simulink library "hmi_udp_lib"  (Simulink 8.2)
settings: Solver=ode1  StartTime=0.0  StopTime=Inf  FixedStep=0.001  RelTol=1e-3
PostLoadFcn:
  | , if any(exist('dsrtsu_mdlpostloadfcn', 'file') == [2, 3, 6]), try dsrtsu_mdlpostloadfcn('Execute', bdroot); catch fprintf('Error in PostLoadFcn (dsrtsu_mdlpostloadfcn) for model "%s":\n %s\n', bdroot, lasterr); end, end,
undefined symbols (not defined in the file): XXX
libraries: rtiethernetudplib x2, parse_utils x1
settings Model: DSRTSU_INTERNAL_RTI_VER=450  DSRTSU_INTERNAL_RTI_TYPE=rti1401  DSRTSU_INTERNAL_RTIFPGA=40  Creator=rushk1  LastModifiedBy=rushk1

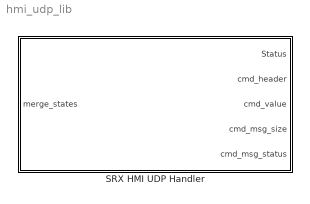
== system hmi_udp_lib ==
  SRX HMI UDP Handler : Subsystem

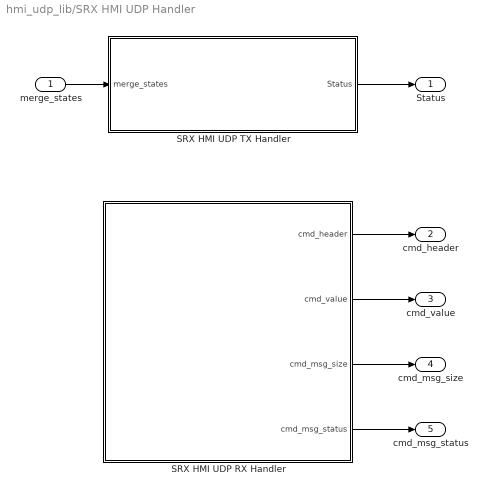
== system hmi_udp_lib/SRX HMI UDP Handler ==
  merge_states : Inport
  SRX HMI UDP RX Handler : Subsystem
  SRX HMI UDP TX Handler : Subsystem
  Status : Outport
  cmd_header : Outport  Port=2
  cmd_value : Outport  Port=3
  cmd_msg_size : Outport  Port=4
  cmd_msg_status : Outport  Port=5
  wires:
  SRX HMI UDP TX Handler/1(Status) -> Status/1
  merge_states/1 -> SRX HMI UDP TX Handler/1(merge_states)
  SRX HMI UDP RX Handler/4(cmd_msg_status) -> cmd_msg_status/1
  SRX HMI UDP RX Handler/3(cmd_msg_size) -> cmd_msg_size/1
  SRX HMI UDP RX Handler/2(cmd_value) -> cmd_value/1
  SRX HMI UDP RX Handler/1(cmd_header) -> cmd_header/1

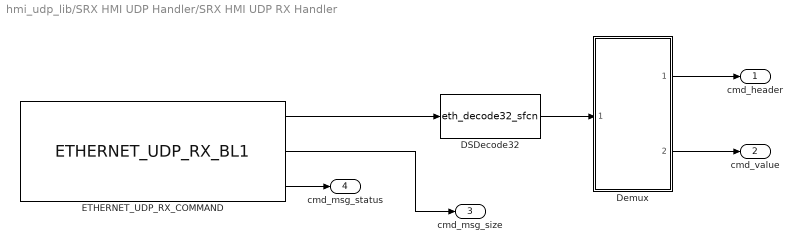
== system hmi_udp_lib/SRX HMI UDP Handler/SRX HMI UDP RX Handler ==
  "DSDecode32 " : S-Function  FunctionName=eth_decode32_sfcn  Parameters=byteordering,offset,auto_offset,datatype,one_datatype,sampletime  EnableBusSupport=off  mask(DSDecode32){byteordering=big endian (Motorola), offset=[0], auto_offset=on, datatype=[3,3], one_datatype=off, sampletime=-1}
      mask prompts: byteordering "Byte ordering:"; offset "Offset (bytes):"; auto_offset "Auto offset"; one_datatype "One datatype only"
      mask help:
      | Converts a 32bit WORD input data stream into the specified datatypes on the output port.
      |
      | Datatype Codes:
      | BOOLEAN:  1   //   INT8      :  2    //   UINT8    :  3
      | INT16       :  4   //   UINT16 :  5    //   INT32     :  6
      | UINT32    :  7   //   FLOAT   :  8    //   DOUBLE:  9
      mask Help:
      | The 'DSDecode32' block allows to decode an UInt32 vector containing encoded elements of various data types to an output vector of double values. It is intended to use this block in conjunction with the 'DS4504_ETH_Receive' block which delivers this format as data output. Data received from the Ethernet via the 'DS4504_ETH_Receive' block is performed in Intel byte order ('Little Endian').
      | 
      | <br>
      | <br>
      | 
      | <h2>Parameters</h2>
      | <br>
      | <br>
      | 
      | <b>Byte ordering (only relevant for offline simulation)</b>
      | <br>
      | <blockquote>
      | The byte order of the input vector has to be specified. In case of running a real-time application the appropriate byte order (Motorola for DS1005 and Intel for DS1006) is selected automatically. Therefore the byte order setting has no influence on the online simulation.
      | </blockquote>
      | <br>
      | 
      | <b>Offset (bytes)</b>
      | <br>
      | <blockquote>
      | This is for defining a vector of offsets which specifies the position of each element within the input vector. The offsets must be entered as an array (e.g. [1 10 . 50 54] ) using the same order as for the corresponding data type vector (see (4)). This option is useful if you have gaps between adjacent elements.
      | </blockquote>
      | <br>
      | 
      | <b>Auto offset</b>
      | <br>
      | <blockquote>
      | When activating this checkbox parameter, the edit field 'Offset' is disabled and the byte offsets in the input vector are calculated automatically concerning the specified data types (no gaps presupposed). Any previous setting in the offset vector would be ignored.
      | </blockquote>
      | <br>
      | 
      | <b>Datatype</b>
      | <br>
      | <blockquote>
      | This is for defining a vector of data types which specifies the type for each element in the input vector. Supported data types are Boolean, Int8, UInt8, Int16, UInt16, Int32, UInt32, Float and Double, which are determined by using the corresponding data type codes shown in the following table:
      | <br>
      | <br>
      | <table BORDER=1 ALIGN="center">
      | <TR>
      | <TH WIDTH=20%>Data type</TH>
      | <TH WIDTH=20%>Data type code</TH>
      | <TH WIDTH=20%>Length in bytes</TH>
      | </TR>
      | <TR><TD>Boolean</TD><TD ALIGN="center">1</TD><TD ALIGN="center">1</TD></TR>
      | <TR><TD>Int8</TD><TD ALIGN="center">2</TD><TD ALIGN="center">1</TD></TR>
      | <TR><TD>Uint8</TD><TD ALIGN="center">3</TD><TD ALIGN="center">1</TD></TR>
      | <TR><TD>Int16</TD><TD ALIGN="center">4</TD><TD ALIGN="center">2</TD></TR>
      | <TR><TD>Uint16</TD><TD ALIGN="center">5</TD><TD ALIGN="center">2</TD></TR>
      | <TR><TD>Int32</TD><TD ALIGN="center">6</TD><TD ALIGN="center">4</TD></TR>
      | <TR><TD>Uint32</TD><TD ALIGN="center">7</TD><TD ALIGN="center">4</TD></TR>
      | <TR><TD>Float</TD><TD ALIGN="center">8</TD><TD ALIGN="center">4</TD></TR>
      | <TR><TD>Double</TD><TD ALIGN="center">9</TD><TD ALIGN="center">8</TD></TR>
      | </TABLE>
      | </blockquote>
      | <br>
      | 
      | <b>One datatype only</b>
      | <br>
      | <blockquote>
      | This option is useful if all elements of the input vector have the same data type. If the checkbox is activated the first element of the data type vector specifies the data type to be used. In this case it is naturally sufficient to enter only one number which applies for the complete input vector.
      | </blockquote>
      | <br>
      | 
      | <b>Sample time</b>
      | <br>
      | <blockquote>
      | The desired sample time for this block has to be entered here. Alternatively it can be  inherited from the Simulink model by using '-1'.
      | </blockquote>
      | <br>
      mask TypeOptions byteordering: big endian (Motorola) | little endian (Intel)
      mask Display: text(0.5,0.5,'DSDecode32','HorizontalAlignment','center')
  Demux : Subsystem
  ETHERNET_UDP_RX_COMMAND : rtiethernetudplib/ETHERNET_UDP_RX_BL1  InterfaceName=NOT SPECIFIED  BoardType=ETH Type 1  ModuleNo=1  ChannelNo=1  SocketNo=4  MaxMessageSize=5  LocalSocket=XXX.XXX.XXX.XXX:5000  RemoteSocket=XXX.XXX.XXX.XXX:5000  DSProperties=struct('RTI',struct('Version',uint32(1),'BlockType',struct('isSLSource',uint8(1),'isSLSink',uint8(0),'isHWSource',uint8(0),'isHWSink',uint8(1),'isSetup',uint8(0),'isInline',uint8(1),'isNonInline',uint8(1),'isInterrupt',uint8(0),'isChannelwise',uint8(1)),'IOBoardType','DSETHERNETUDP','UnitType','ETHUDP','Identifier','RX','DialogType','SL','BlockSet','RTIETHERNETUDP','SlaveProcessor','NONE'))  RTIBlockInterface=struct('OutputPortsWidth',int32([1 1 1]),'OutputPortsActive',[1 1 1],'OutputPortsName',{{'Data',['Message Size'],'Status'}},'OutputPortsDataType',{{'SS_UINT32','SS_INT32','SS_BOOLEAN'}},'BlockDisplay',{{['Ethernet UDP Receive\nBoard Type: ETH Type 1\nModule: 1\nSocket: 4\nMaximum Message Size: 5'],'center'}},'IconTransparency','on','InitLevel',3,'BlockName',struct('Token',{{'ETHERNET_UDP_RX_BL1'}}),'MaskDescription',['To receive messages from the Ethernet UDP interface.'])  RTIBlockParameters=struct('InterfaceName',{{['NOT SPECIFIED'],'OFF',[]}},'BoardType',{{1,'OFF',[]}},'ModuleNo',{{1,'OFF',[1 16]}},'ChannelNo',{{1,'OFF',[1 2]}},'SocketNo',{{4,'OFF',[1 4]}},'MaxMessageSize',{{5,'ON',[1 1472]}},'LocalSocket',{{'XXX.XXX.XXX.XXX:5000','OFF',[]}},'RemoteSocket',{{'XXX.XXX.XXX.XXX:5000','OFF',[]}})  RTISFcnParameters=struct('InterfaceName','char','BoardType','double','ModuleNo','double','ChannelNo','double','SocketNo','double','MaxMessageSize','double','LocalSocket','char','RemoteSocket','char')  RTIBlockParaDefault=struct('InterfaceName','rti_ethernet_interface_name','BoardType',1,'ModuleNo',1,'ChannelNo',1,'SocketNo',1,'MaxMessageSize',625,'LocalSocket','XXX.XXX.XXX.XXX:5000','RemoteSocket','XXX.XXX.XXX.XXX:5000')
  cmd_header : Outport
  cmd_value : Outport  Port=2
  cmd_msg_size : Outport  Port=3
  cmd_msg_status : Outport  Port=4
  wires:
  ETHERNET_UDP_RX_COMMAND/1 -> "DSDecode32 "/1
  ETHERNET_UDP_RX_COMMAND/3 -> cmd_msg_status/1
  ETHERNET_UDP_RX_COMMAND/2 -> cmd_msg_size/1
  "DSDecode32 "/1 -> Demux/1(cmd_msg)
  Demux/1(cmd_header) -> cmd_header/1
  Demux/2(cmd_ value) -> cmd_value/1

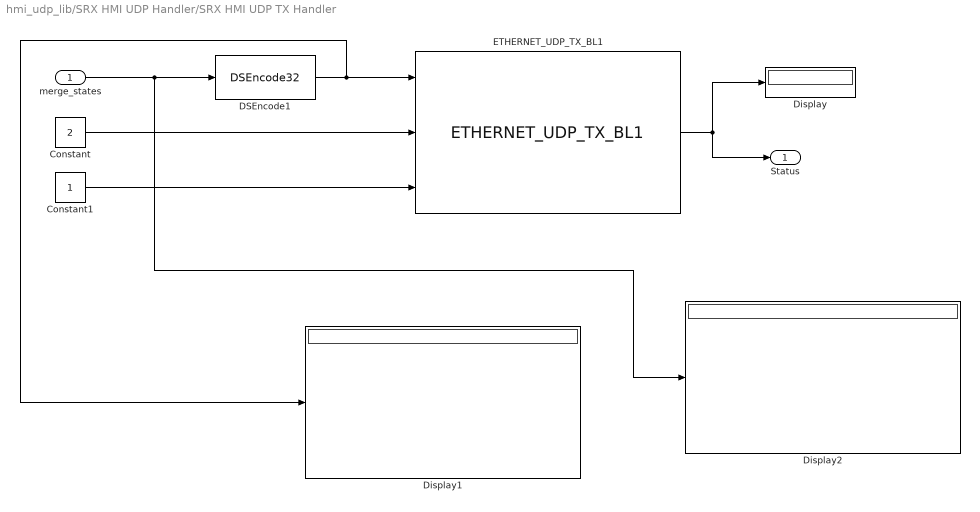
== system hmi_udp_lib/SRX HMI UDP Handler/SRX HMI UDP TX Handler ==
  merge_states : Inport
  Constant : Constant  Value=2  OutDataTypeStr=int32
  Constant1 : Constant  OutDataTypeStr=boolean
  DSEncode1 : parse_utils/DSEncode32  byteordering=little endian (Intel)  offset=[ 0 ]  auto_offset=on  datatype=[3 3]  one_datatype=off  sampletime=-1
  Display : Display
  Display1 : Display
      settings: Format=binary (Stored Integer)
  Display2 : Display
      settings: Format=binary (Stored Integer)
  ETHERNET_UDP_TX_BL1 : rtiethernetudplib/ETHERNET_UDP_TX_BL1  InterfaceName=NOT SPECIFIED  BoardType=ETH Type 1  ModuleNo=1  ChannelNo=1  SocketNo=4  MaxMessageSize=2  SendTimeout=0.0005  LocalSocket=XXX.XXX.XXX.XXX:5000  RemoteSocket=XXX.XXX.XXX.XXX:5000  DSProperties=struct('RTI',struct('Version',uint32(2),'BlockType',struct('isSLSource',uint8(1),'isSLSink',uint8(1),'isHWSource',uint8(1),'isHWSink',uint8(1),'isSetup',uint8(0),'isInline',uint8(1),'isNonInline',uint8(1),'isInterrupt',uint8(0),'isChannelwise',uint8(1)),'IOBoardType','DSETHERNETUDP','UnitType','ETHUDP','Identifier','TX','DialogType','SL','BlockSet','RTIETHERNETUDP','SlaveProcessor','NONE'))  RTIBlockInterface=struct('OutputPortsWidth',int32(1),'OutputPortsActive',1,'OutputPortsName',{{'Status'}},'OutputPortsDataType',{{'SS_UINT16'}},'InputPortsWidth',int32([1 1 1]),'InputPortsActive',[1 1 1],'InputPortsName',{{'Data',['Message Size'],'Enable'}},'InputPortsDataType',{{'SS_UINT32','SS_INT32','SS_BOOLEAN'}},'BlockDisplay',{{['Ethernet UDP Transmit\nBoard Type: ETH Type 1\nModule: 1\nSocket: 4\nMaximum Message Size: 2'],'center'}},'IconTransparency','on','InitLevel',3,'BlockName',struct('Token',{{'ETHERNET_UDP_TX_BL1'}}),'MaskDescription',['To send messages via the Ethernet UDP interface.'])  RTIBlockParameters=struct('InterfaceName',{{['NOT SPECIFIED'],'OFF',[]}},'BoardType',{{1,'OFF',[]}},'ModuleNo',{{1,'OFF',[1 16]}},'ChannelNo',{{1,'OFF',[1 2]}},'SocketNo',{{4,'OFF',[1 4]}},'MaxMessageSize',{{2,'ON',[1 1472]}},'SendTimeout',{{0.0005,'ON',[1e-05 2]}},'LocalSocket',{{'XXX.XXX.XXX.XXX:5000','OFF',[]}},'RemoteSocket',{{'XXX.XXX.XXX.XXX:5000','OFF',[]}})  RTISFcnParameters=struct('InterfaceName','char','BoardType','double','ModuleNo','double','ChannelNo','double','SocketNo','double','MaxMessageSize','double','SendTimeout','double','LocalSocket','char','RemoteSocket','char')  RTIBlockParaDefault=struct('InterfaceName','rti_ethernet_interface_name','BoardType',1,'ModuleNo',1,'ChannelNo',1,'SocketNo',1,'MaxMessageSize',625,'SendTimeout',0.0005,'LocalSocket','XXX.XXX.XXX.XXX:5000','RemoteSocket','XXX.XXX.XXX.XXX:5000')
  Status : Outport
  wires:
  ETHERNET_UDP_TX_BL1/1 -> Status/1, Display/1
  Constant1/1 -> ETHERNET_UDP_TX_BL1/3
  Constant/1 -> ETHERNET_UDP_TX_BL1/2
  DSEncode1/1 -> Display1/1, ETHERNET_UDP_TX_BL1/1
  merge_states/1 -> Display2/1, DSEncode1/1

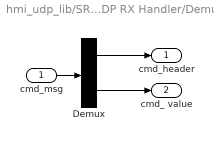
== system hmi_udp_lib/SRX HMI UDP Handler/SRX HMI UDP RX Handler/Demux ==
  cmd_msg : Inport
  Demux : Demux  Outputs=2
  cmd_header : Outport
  cmd_ value : Outport  Port=2
  wires:
  cmd_msg/1 -> Demux/1
  Demux/1 -> cmd_header/1
  Demux/2 -> cmd_ value/1
